simulink model "OPC_AUTOMATIZACIO_PROCESOS"  (R2014b)
settings: Solver=ode45  StartTime=0.0  StopTime=inf  RelTol=1e-3
libraries: opclib x5
settings Model: Creator=user  LastModifiedBy=CONTROL02

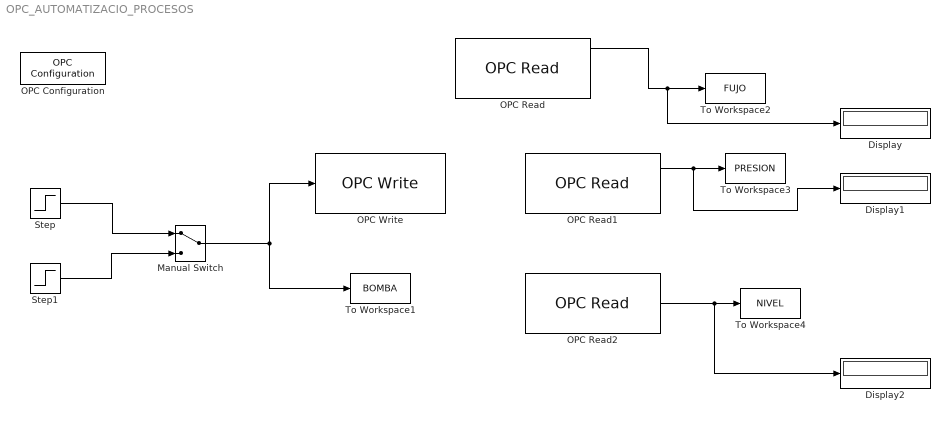
== system OPC_AUTOMATIZACIO_PROCESOS ==
  Display : Display
  Display1 : Display
  Display2 : Display
  Manual Switch : ManualSwitch
  OPC Configuration : opclib/OPC Configuration  opcServers=localhost/Kepware.KEPServerEX.V6/10  errMissingItems=Error  errReadWrite=Warn  errShutdown=Error  errRTViolation=Warn  rtEnable=on  speedup=1  showLatency=off  beingUsed=on
  OPC Read : opclib/OPC Read  serverHost=localhost  serverID=Kepware.KEPServerEX.V6  itemIDs=1500.Device1.FLUJO  readMode=Synchronous (cache)  dataType=double  updateRate=0.5  showQual=on  showTS=on  tsMode=Seconds since start
  OPC Read1 : opclib/OPC Read  serverHost=localhost  serverID=Kepware.KEPServerEX.V6  itemIDs=1500.Device1.PRESION  readMode=Synchronous (cache)  dataType=double  updateRate=0.5  showQual=off  showTS=on  tsMode=Seconds since start
  OPC Read2 : opclib/OPC Read  serverHost=localhost  serverID=Kepware.KEPServerEX.V6  itemIDs=1500.Device1.NIVEL  readMode=Synchronous (cache)  dataType=double  updateRate=0.5  showQual=off  showTS=off  tsMode=Seconds since start
  OPC Write : opclib/OPC Write  serverHost=localhost  serverID=Kepware.KEPServerEX.V6  itemIDs=1500.Device1.BOMBA  writeMode=Synchronous  updateRate=0
  Step : Step  Time=0  After=20000  SampleTime=0
  Step1 : Step  Time=0  After=0  SampleTime=0
  To Workspace1 : ToWorkspace  VariableName=BOMBA  SampleTime=-1
  To Workspace2 : ToWorkspace  VariableName=FUJO  SampleTime=-1
  To Workspace3 : ToWorkspace  VariableName=PRESION  SampleTime=-1
  To Workspace4 : ToWorkspace  VariableName=NIVEL  SampleTime=-1
  wires:
  Manual Switch/1 -> OPC Write/1, To Workspace1/1
  Step/1 -> Manual Switch/1
  Step1/1 -> Manual Switch/2
  OPC Read/1 -> Display/1, To Workspace2/1
  OPC Read1/1 -> Display1/1, To Workspace3/1
  OPC Read2/1 -> Display2/1, To Workspace4/1
